simulink model "robotModel"  (R2024a)
settings: Solver=VariableStepAuto  StartTime=0.0  StopTime=10.0  RelTol=1e-3
InitFcn:
  | modelParamsDD = Simulink.data.dictionary.open('modelConfigData.sldd');
  | sectModel = getSection(modelParamsDD,'Design Data');
  | controlRateTemp = getValue(getEntry(sectModel,'controlRate'));
  | 
  | motorParamsDD = Simulink.data.dictionary.open('motorParametersData.sldd');
  | robotParamsDD = Simulink.data.dictionary.open('robotModelData.sldd');
  | controlParamsDD = Simulink.data.dictionary.open('controlVariablesData.sldd');
  | sectMotor = getSection(motorParamsDD,'Design Data');
  | sectRobot = getSection(robotParamsDD,'Design Data');
  | sectControl = getSection(controlParamsDD,'Design Data');
  | 
  | % Physical Parameters
  | % M = getValue(getEntry(sectRobot,'massOfCart'));    % mass of cart
  | M = 1;
  | m = 1;
  | % m = getValue(getEntry(sectRobot,'massOfPendulum'));    % mass of pendulum
  | % L = getValue(getEntry(sectRobot,'lengthToPendulumCenterOfMass'));    % length to pendulum center of mass
  | L = 2;
  | g = 9.81;   % gravity
  | I = getValue(getEntry(sectRobot,'inertiaOfPendulum'));  % inertia of pendulum
  | r = getValue(getEntry(sectRobot,'wheelRadius'));   % 5 cm wheel radius
  | 
  | % Servo motor state: i, omega
  | R_m = getValue(getEntry(sectMotor,'armatureResistance')); % motor resistance
  | L_m = getValue(getEntry(sectMotor,'armatureInductance')); % motor coil inductance
  | K_m = getValue(getEntry(sectMotor,'motorTorqueConstantKm')); % motor torque constant
  | K_b = getValue(getEntry(sectMotor,'backEMFConstantKb')); % motor electrical consant
  | K_f = getValue(getEntry(sectMotor,'viscousFriction')); % viscous friction
  | J = getValue(getEntry(sectMotor,'motorInertia'));  % inertia of rotor
  | 
  | maxVoltage = 12;
settings Model: Creator=Peter  LastModifiedBy=Peter
settings DataIOCC: SaveOutput=off  SaveTime=off

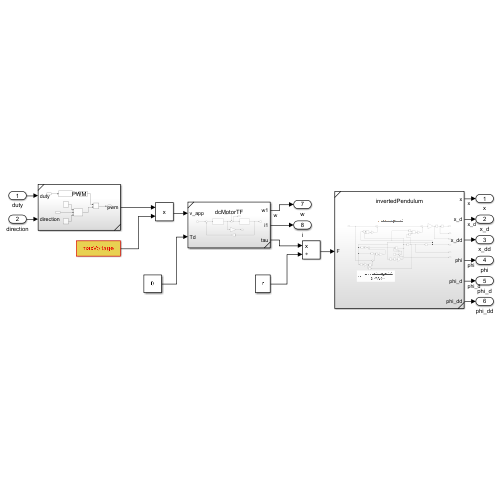
[thumbnail: Simulink's stored preview of the top-level diagram]
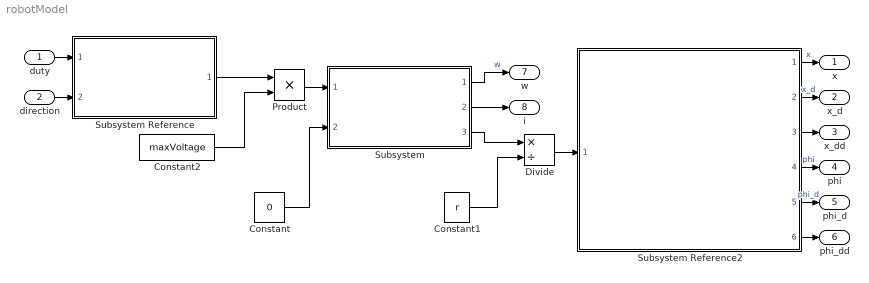
== system robotModel ==
  duty : Inport  OutDataTypeStr=single  PortDimensions=1
  direction : Inport  Port=2  OutDataTypeStr=int8  PortDimensions=1
  Constant : Constant  Value=0
  Constant1 : Constant  Value=r
  Constant2 : Constant  Value=maxVoltage
  Divide : Product  Inputs=*/
  Product : Product
  Subsystem : Subsystem  ReferencedSubsystem=dcMotorTF
  Subsystem Reference : Subsystem  ReferencedSubsystem=PWM
  Subsystem Reference2 : Subsystem  ReferencedSubsystem=invertedPendulum
  x : Outport  OutDataTypeStr=double  PortDimensions=1  SampleTime=0
  x_d : Outport  Port=2  OutDataTypeStr=double  PortDimensions=1  SampleTime=0
  x_dd : Outport  Port=3  OutDataTypeStr=double  PortDimensions=1  SampleTime=0
  phi : Outport  Port=4  OutDataTypeStr=double  PortDimensions=1  SampleTime=0
  phi_d : Outport  Port=5  OutDataTypeStr=double  PortDimensions=1  SampleTime=0
  phi_dd : Outport  Port=6  OutDataTypeStr=double  PortDimensions=1  SampleTime=0
  w : Outport  Port=7  OutDataTypeStr=double  PortDimensions=1  SampleTime=0
  i : Outport  Port=8  OutDataTypeStr=double  PortDimensions=1  SampleTime=0
  wires:
  Constant1/1 -> Divide/2
  Divide/1 -> Subsystem Reference2/1
  Subsystem Reference/1 -> Product/1
  Subsystem Reference2/4 -> phi/1  "phi"
  Subsystem Reference2/1 -> x/1  "x"
  Subsystem Reference2/5 -> phi_d/1  "phi_d"
  duty/1 -> Subsystem Reference/1
  Subsystem Reference2/2 -> x_d/1  "x_d"
  Subsystem/1 -> w/1  "w"
  direction/1 -> Subsystem Reference/2
  Subsystem/3 -> Divide/1
  Subsystem/2 -> i/1
  Subsystem Reference2/6 -> phi_dd/1
  Subsystem Reference2/3 -> x_dd/1
  Constant/1 -> Subsystem/2
  Product/1 -> Subsystem/1
  Constant2/1 -> Product/2
